simulink model "minvalid_subsys"  (Simulink 8.0)
settings: Solver=ode45  StartTime=0.0  StopTime=10.0  RelTol=1e-3
libraries: mblibv1 x1
settings Model: FPTRunName=Active  Creator=mshakeri  LastModifiedBy=mtocci  ExtModeAutoUpdateStatusClock=off
settings DataIOCC: SignalLoggingSaveFormat=ModelDataLogs
settings OptimizationCC: InlineParams=on  InitFltsAndDblsToZero=on  EfficientMapNaN2IntZero=off
settings DebuggingCC: SaveWithParameterizedLinksMsg=none  SignalResolutionControl=TryResolveAllWithWarning  MultiTaskDSMMsg=warning  MultiTaskCondExecSysMsg=none  SigSpecEnsureSampleTimeMsg=none  FcnCallInpInsideContextMsg=Use local settings  StrictBusMsg=None
settings SFSimCC: SimParseCustomCode=off
settings RTWCC: IncludeERTFirstTime=on
settings GRTTargetCC: TargetFcnLib=ansi_tfl_tmw.mat  CombineOutputUpdateFcns=off
settings ConfigurationSet: Description=SimMechanicsII  OpenEditorOnUpdate=on
settings DiagnosticsConfigSet: RedundantConstraints=warning  UnstableConstraints=warning  InvalidFilename=error  InvalidUnit=error  InvalidDimension=error  RangeError=error  InvalidJoint=error  InvalidPrimitive=error  InvalidTarget=error  FloatingEntity=warning  FloatingImporterExporter=warning  DanglingBlock=warning  UnconnectedTransformSensorFramePort=warning  RedundantBlock=warning  ShortedTransform=error  RigidCycle=error  ConflictingRefFrames=error  ConflictingMachineEnvironments=error  RigidlyBoundJoint=error

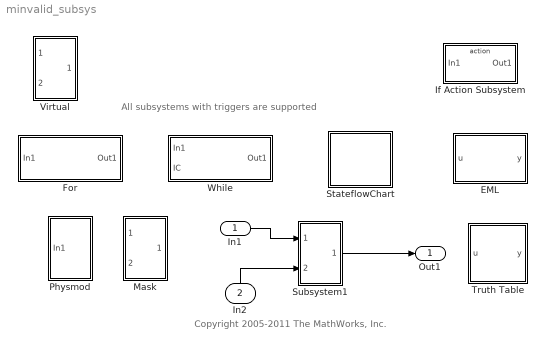
== system minvalid_subsys ==
  note: Copyright 2005-2011 The MathWorks, Inc.
  note: All subsystems with triggers are supported
  In1 : Inport
  In2 : Inport  Port=2
  EML : Stateflow chart  TreatAsAtomicUnit=on
  For : Subsystem  TreatAsAtomicUnit=on
  If Action Subsystem : Subsystem  TreatAsAtomicUnit=on
  Mask : Subsystem  TreatAsAtomicUnit=on  mask{k=0}
      mask prompts: k "myGain"
  Physmod : Subsystem
  StateflowChart : Stateflow chart  TreatAsAtomicUnit=on
  Subsystem1 : Subsystem  mask{k=0}
      mask prompts: k "subsysGain"
  Truth Table : Stateflow chart  TreatAsAtomicUnit=on
  Virtual : Subsystem
  While : Subsystem  TreatAsAtomicUnit=on
  Out1 : Outport
  wires:
  In1/1 -> Subsystem1/1(In1)
  Subsystem1/1(Out1) -> Out1/1
  In2/1 -> Subsystem1/2(In2)

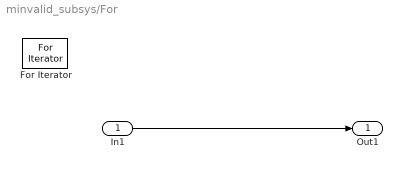
== system minvalid_subsys/For ==
  In1 : Inport
  For Iterator : ForIterator
  Out1 : Outport
  wires:
  In1/1 -> Out1/1

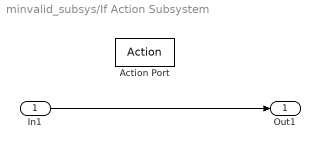
== system minvalid_subsys/If Action Subsystem ==
  In1 : Inport
  Action Port : ActionPort
  Out1 : Outport
  wires:
  In1/1 -> Out1/1

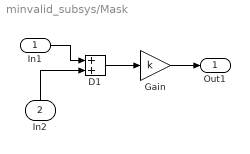
== system minvalid_subsys/Mask ==
  In1 : Inport
  In2 : Inport  Port=2
  D1 : Sum  SaturateOnIntegerOverflow=on  InputSameDT=on  OutDataTypeStr=Inherit: Same as first input
  Gain : Gain  Gain=k
  Out1 : Outport
  wires:
  In1/1 -> D1/1
  Gain/1 -> Out1/1
  In2/1 -> D1/2
  D1/1 -> Gain/1

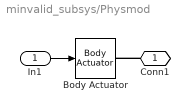
== system minvalid_subsys/Physmod ==
  In1 : Inport
  Body Actuator : mblibv1/Sensors &  Actuators/Body Actuator  UpdateFromCAD=off  PhysicalDomain=Mechanical  PortType=blob  ActuationStyle=Force  AngleUnits=deg  ArcVelocityUnits=deg/s  ArcAccelerationUnits=deg/s^2  CoordPositionUnits=m  VelocityUnits=m/s  AccelerationUnits=m/s^2  ForceUnits=N  TorqueUnits=N-m  ActiveIO=off  Width=1  DialogClass=MechanicalActuatorBlock  ReferenceFrame=Absolute (World)  Angle=off  CoordPosition=on  Force=on  Torque=off
  Conn1 : PMIOPort  Port=1  Side=Right
  wires:
  In1/1 -> Body Actuator/1
  connections:
  Conn1/RConn1 -- Body Actuator/RConn1

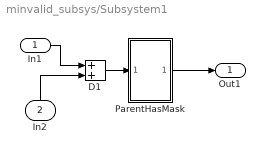
== system minvalid_subsys/Subsystem1 ==
  In1 : Inport
  In2 : Inport  Port=2
  D1 : Sum  SaturateOnIntegerOverflow=on  InputSameDT=on  OutDataTypeStr=Inherit: Same as first input
  ParentHasMask : Subsystem  TreatAsAtomicUnit=on
  Out1 : Outport
  wires:
  ParentHasMask/1(Out1) -> Out1/1
  In1/1 -> D1/1
  In2/1 -> D1/2
  D1/1 -> ParentHasMask/1(In1)

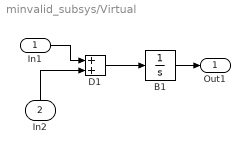
== system minvalid_subsys/Virtual ==
  In1 : Inport
  In2 : Inport  Port=2
  B1 : Integrator
  D1 : Sum  SaturateOnIntegerOverflow=on  InputSameDT=on  OutDataTypeStr=Inherit: Same as first input
  Out1 : Outport
  wires:
  D1/1 -> B1/1
  In2/1 -> D1/2
  B1/1 -> Out1/1
  In1/1 -> D1/1

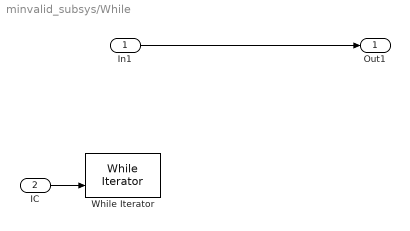
== system minvalid_subsys/While ==
  In1 : Inport
  IC : Inport  Port=2
  While Iterator : WhileIterator
  Out1 : Outport
  wires:
  IC/1 -> While Iterator/2
  In1/1 -> Out1/1

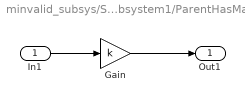
== system minvalid_subsys/Subsystem1/ParentHasMask ==
  In1 : Inport
  Gain : Gain  Gain=k
  Out1 : Outport
  wires:
  In1/1 -> Gain/1
  Gain/1 -> Out1/1

== stateflow chart StateflowChart ==

== matlab function EML ==
  data: u input double; y output double
function y = fcn(u)
% This block supports an embeddable subset of the MATLAB language.
% See the help menu for details. 

y = u;

== matlab function Truth Table ==
  data: u input double; y output double
function y = fcn(u)

aVarTruthTableCondition_1 = false;
aVarTruthTableCondition_2 = false;


% Example condition 1

aVarTruthTableCondition_1 = logical(u >= 0);

% Example condition 2

aVarTruthTableCondition_2 = logical(u ^ 2 <= 1);

if (aVarTruthTableCondition_1 && aVarTruthTableCondition_2)
    aFcnTruthTableAction_1();
elseif (~aVarTruthTableCondition_1 && ~aVarTruthTableCondition_2)
    aFcnTruthTableAction_1();
else % Default
    aFcnTruthTableAction_2();
end

function aFcnTruthTableAction_1()

% Example action 1 called from D1 & D2 column in condition table

y = u;

function aFcnTruthTableAction_2()

% Example action 2 called from D3 column in condition table

y = 1 / u;
